simulink model "CIOBAN_AnaMaria_pendul"  (R2025a)
settings: Solver=FixedStepAuto  StartTime=0.0  StopTime=Tfin  FixedStep=Ts  RelTol=1e-3
values from neighbouring files (symbols this model uses):
  b = 0.3+m/24    (= 0.466666666667)    [CIOBAN_AnaMaria_setup_pendul.m]    (also in pendulum_system_setup.m)
  c1 = 180/pi    (= 57.2957795131)    [CIOBAN_AnaMaria_setup_pendul.m]    (also in pendulum_system_setup.m)
  c2 = 4+n/2    (= 9)    [CIOBAN_AnaMaria_setup_pendul.m]    (also in pendulum_system_setup.m)
  delta = 0.125    [CIOBAN_AnaMaria_setup_pendul.m]    (also in pendulum_system_setup.m)
  g = 9.81    [CIOBAN_AnaMaria_setup_pendul.m]    (also in pendulum_system_setup.m)
  l = 1.2-m/24    (= 1.03333333333)    [CIOBAN_AnaMaria_setup_pendul.m]    (also in pendulum_system_setup.m)
  M = 0.8-n/48    (= 0.591666666667)    [CIOBAN_AnaMaria_setup_pendul.m]    (also in pendulum_system_setup.m)
  meas_rep = round(7+n/2)    [CIOBAN_AnaMaria_setup_pendul.m]    (also in pendulum_system_setup.m)
  t1 = 20    [CIOBAN_AnaMaria_setup_pendul.m]    (also in pendulum_system_setup.m)
  Ts = 500e-6    (= 0.0005)    [CIOBAN_AnaMaria_setup_pendul.m]    (also in pendulum_system_setup.m)
  u_star = 1.2+n*0.075    (= 1.95)    [CIOBAN_AnaMaria_setup_pendul.m]    (also in pendulum_system_setup.m)
  umax = 5    [CIOBAN_AnaMaria_setup_pendul.m]    (also in pendulum_system_setup.m)
  umin = -5    [CIOBAN_AnaMaria_setup_pendul.m]    (also in pendulum_system_setup.m)
  whtn_pow_in = 1e-10*(Ts*1e4)/2    (= 2.5e-10)    [CIOBAN_AnaMaria_setup_pendul.m]    (also in pendulum_system_setup.m)
  whtn_pow_out = 1e-3*Ts    (= 5e-07)    [CIOBAN_AnaMaria_setup_pendul.m]    (also in pendulum_system_setup.m)
  whtn_seed_in = 23341+m+2*n    (= 23365)    [CIOBAN_AnaMaria_setup_pendul.m]    (also in pendulum_system_setup.m)
  whtn_seed_out = 23342-m-2*n    (= 23318)    [CIOBAN_AnaMaria_setup_pendul.m]    (also in pendulum_system_setup.m)
  whtn_Ts_in = Ts*2    (= 0.001)    [CIOBAN_AnaMaria_setup_pendul.m]    (also in pendulum_system_setup.m)
  whtn_Ts_out = Ts*2    (= 0.001)    [CIOBAN_AnaMaria_setup_pendul.m]    (also in pendulum_system_setup.m)
  x0_slx = [(n+3)/50,(-1)^(n+1)*m/20]    [CIOBAN_AnaMaria_setup_pendul.m]    (also in pendulum_system_setup.m)
  ymax = 100    [CIOBAN_AnaMaria_setup_pendul.m]    (also in pendulum_system_setup.m)
  ymin = -100    [CIOBAN_AnaMaria_setup_pendul.m]    (also in pendulum_system_setup.m)
undefined symbols (not defined in the file or in its folder): t0
libraries: simulink x2
settings Model: Creator=mircea  LastModifiedBy=ana

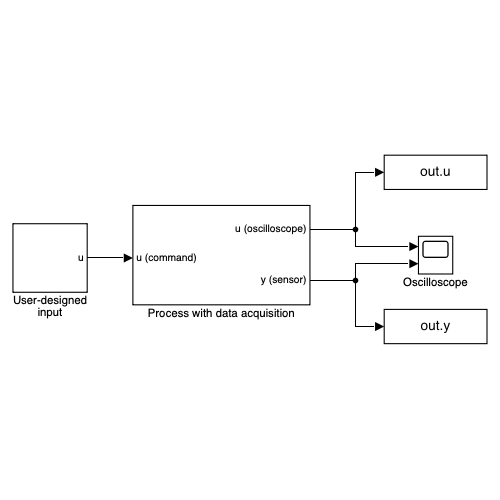
[thumbnail: Simulink's stored preview of the top-level diagram]
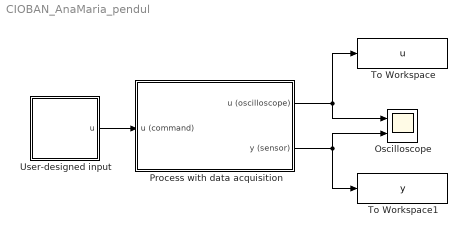
== system CIOBAN_AnaMaria_pendul ==
  Oscilloscope : Scope  NumInputPorts=2
      settings: ActiveDisplayYMinimum=-18.75  ActiveDisplayYMaximum=18.75
  Process with data acquisition : Subsystem
  To Workspace : ToWorkspace  VariableName=u  SampleTime=Ts
  To Workspace1 : ToWorkspace  VariableName=y  SampleTime=Ts
  User-designed input : Subsystem
  wires:
  Process with data acquisition/1(u (oscilloscope)) -> Oscilloscope/1, To Workspace/1
  Process with data acquisition/2(y (sensor)) -> Oscilloscope/2, To Workspace1/1
  User-designed input/1(u) -> Process with data acquisition/1(u (command))

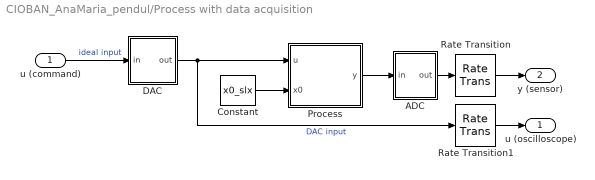
== system CIOBAN_AnaMaria_pendul/Process with data acquisition ==
  u (command) : Inport
  ADC : Subsystem
  Constant : Constant  Value=x0_slx
  DAC : Subsystem
  Process : Subsystem
  Rate Transition : RateTransition  OutPortSampleTime=Ts*meas_rep
  Rate Transition1 : RateTransition  OutPortSampleTime=Ts*meas_rep
  u (oscilloscope) : Outport
  y (sensor) : Outport  Port=2
  wires:
  Constant/1 -> Process/2(x0)
  u (command)/1 -> DAC/1(in)  "ideal input"
  Process/1(y) -> ADC/1(in)
  ADC/1(out) -> Rate Transition/1
  DAC/1(out) -> Process/1(u), Rate Transition1/1  "DAC input"
  Rate Transition/1 -> y (sensor)/1
  Rate Transition1/1 -> u (oscilloscope)/1

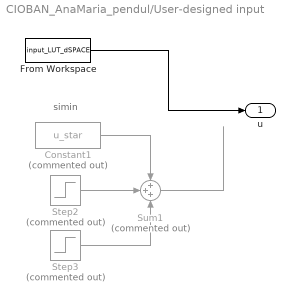
== system CIOBAN_AnaMaria_pendul/User-designed input ==
  note: simin
  Constant1 : Constant  Commented=on  Value=u_star
  From Workspace : FromWorkspace  VariableName=input_LUT_dSPACE  SampleTime=Ts
  Step2 : Step  Commented=on  Time=t0  After=-delta  SampleTime=0
  Step3 : Step  Commented=on  Time=t1  After=2*delta  SampleTime=0
  Sum1 : Sum  Commented=on  Inputs=+++
  u : Outport
  wires:
  Step2/1 -> Sum1/2
  Constant1/1 -> Sum1/1
  Step3/1 -> Sum1/3
  Sum1/1 -> ?
  From Workspace/1 -> u/1

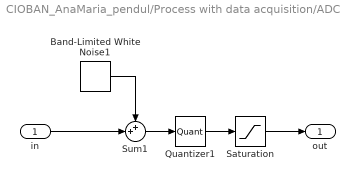
== system CIOBAN_AnaMaria_pendul/Process with data acquisition/ADC ==
  in : Inport
  Band-Limited White Noise1 : simulink/Sources/Band-Limited White Noise  Cov=[whtn_pow_out]  Ts=whtn_Ts_out  seed=[whtn_seed_out]
  Quantizer1 : Quantizer  QuantizationInterval=q_out
  Saturation : Saturate  UpperLimit=ymax  LowerLimit=ymin
  Sum1 : Sum  Inputs=++|
  out : Outport
  wires:
  Quantizer1/1 -> Saturation/1
  Sum1/1 -> Quantizer1/1
  in/1 -> Sum1/2
  Band-Limited White Noise1/1 -> Sum1/1
  Saturation/1 -> out/1

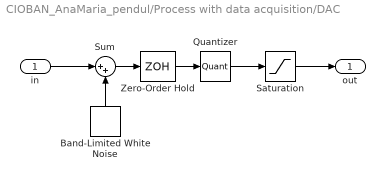
== system CIOBAN_AnaMaria_pendul/Process with data acquisition/DAC ==
  in : Inport
  Band-Limited White Noise : simulink/Sources/Band-Limited White Noise  Cov=[whtn_pow_in]  Ts=whtn_Ts_in  seed=[whtn_seed_in]
  Quantizer : Quantizer  QuantizationInterval=q_in
  Saturation : Saturate  UpperLimit=umax  LowerLimit=umin
  Sum : Sum  Inputs=|++
  Zero-Order Hold : ZeroOrderHold  SampleTime=-1
  out : Outport
  wires:
  Quantizer/1 -> Saturation/1
  Sum/1 -> Zero-Order Hold/1
  in/1 -> Sum/1
  Band-Limited White Noise/1 -> Sum/2
  Zero-Order Hold/1 -> Quantizer/1
  Saturation/1 -> out/1

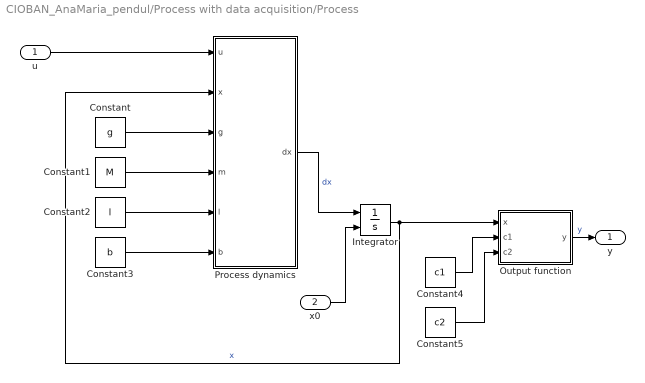
== system CIOBAN_AnaMaria_pendul/Process with data acquisition/Process ==
  u : Inport
  x0 : Inport  Port=2
  Constant : Constant  Value=g
  Constant1 : Constant  Value=M
  Constant2 : Constant  Value=l
  Constant3 : Constant  Value=b
  Constant4 : Constant  Value=c1
  Constant5 : Constant  Value=c2
  Integrator : Integrator  InitialConditionSource=external
  Output function : MATLAB Function  TreatAsAtomicUnit=on
  Process dynamics : MATLAB Function  TreatAsAtomicUnit=on
  y : Outport
  wires:
  u/1 -> Process dynamics/1(u)
  Process dynamics/1(dx) -> Integrator/1  "dx"
  Integrator/1 -> Output function/1(x), Process dynamics/2(x)  "x"
  Output function/1(y) -> y/1  "y"
  x0/1 -> Integrator/2
  Constant/1 -> Process dynamics/3(g)
  Constant1/1 -> Process dynamics/4(m)
  Constant2/1 -> Process dynamics/5(l)
  Constant3/1 -> Process dynamics/6(b)
  Constant4/1 -> Output function/2(c1)
  Constant5/1 -> Output function/3(c2)

== matlab function CIOBAN_AnaMaria_pendul/Process with data acquisition/Process/Process dynamics ==
  data: u input; dx output; x input; g input; m input; l input; b input
function dx = fcn(u,x,g,m,l,b)

Anl = [0,1;0,-b/m/l];
B = [0;1/m/l^2];

dx = Anl*x+B*u+[0;-g/l*sin(x(1))];

== matlab function CIOBAN_AnaMaria_pendul/Process with data acquisition/Process/Output function ==
  data: y output; x input; c1 input; c2 input
function y = fcn(x,c1,c2)

y = [c1,c2]*x;

end
